simulink subsystem "original"  (R2025b)
settings: Solver=VariableStepAuto  StartTime=0.0  StopTime=10.0  RelTol=1e-3
settings Model: Creator=sanborkl  LastModifiedBy=sanborkl

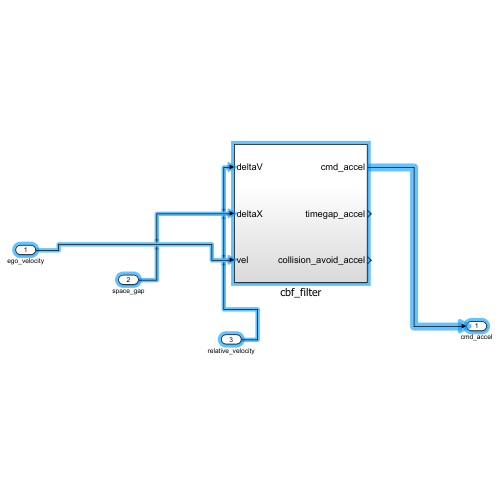
[thumbnail: Simulink's stored preview of the top-level diagram]
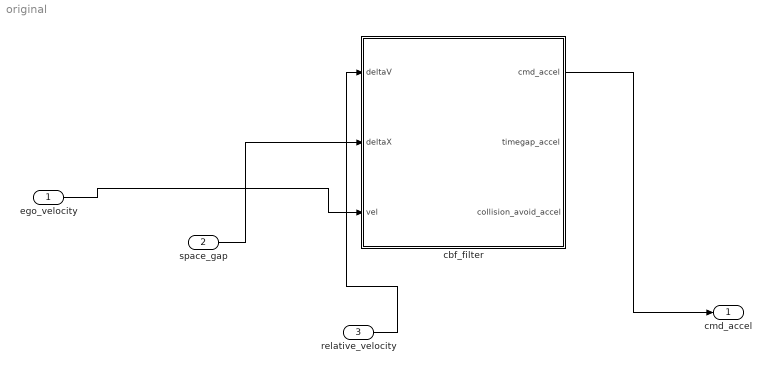
== system original ==
  ego_velocity : Inport
  space_gap : Inport  Port=2
  relative_velocity : Inport  Port=3
  cbf_filter : Subsystem
  cmd_accel : Outport
  wires:
  relative_velocity/1 -> cbf_filter/1(deltaV)
  ego_velocity/1 -> cbf_filter/3(vel)
  space_gap/1 -> cbf_filter/2(deltaX)
  cbf_filter/1(cmd_accel) -> cmd_accel/1

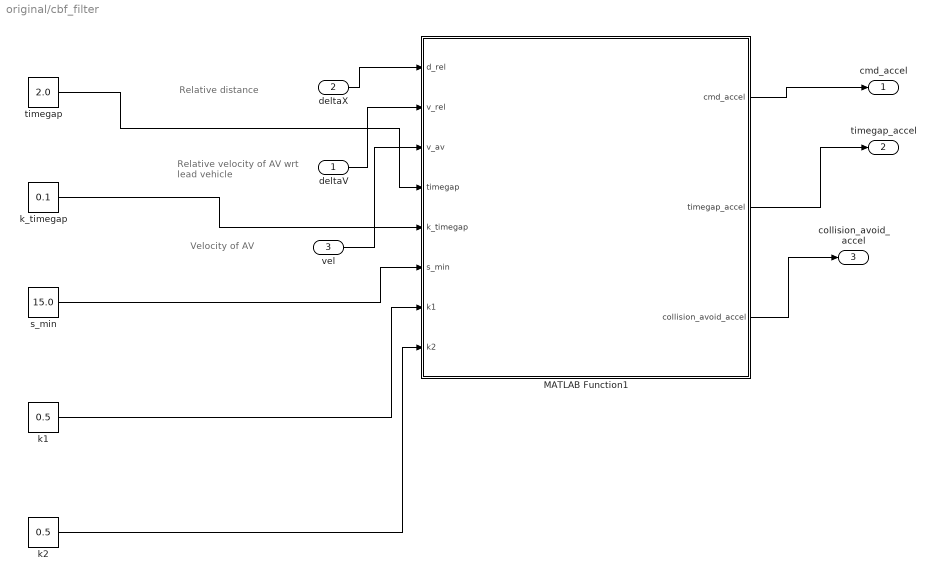
== system original/cbf_filter ==
  note: Velocity of AV
  note: Relative velocity of
      | AV wrt lead vehicle
  note: Relative distance
  deltaV : Inport
  deltaX : Inport  Port=2
  vel : Inport  Port=3
  MATLAB Function1 : MATLAB Function  TreatAsAtomicUnit=on
  k1 : Constant  Value=0.5
  k2 : Constant  Value=0.5
  k_timegap : Constant  Value=0.1
  s_min : Constant  Value=15.0
  timegap : Constant  Value=2.0
  cmd_accel : Outport
  timegap_accel : Outport  Port=2
  collision_avoid_accel : Outport  Port=3
  wires:
  k1/1 -> MATLAB Function1/7(k1)
  timegap/1 -> MATLAB Function1/4(timegap)
  k_timegap/1 -> MATLAB Function1/5(k_timegap)
  s_min/1 -> MATLAB Function1/6(s_min)
  MATLAB Function1/2(timegap_accel) -> timegap_accel/1
  MATLAB Function1/1(cmd_accel) -> cmd_accel/1
  vel/1 -> MATLAB Function1/3(v_av)
  deltaV/1 -> MATLAB Function1/2(v_rel)
  deltaX/1 -> MATLAB Function1/1(d_rel)
  k2/1 -> MATLAB Function1/8(k2)
  MATLAB Function1/3(collision_avoid_accel) -> collision_avoid_accel/1

== matlab function original/cbf_filter/MATLAB Function1 ==
  data: cmd_accel output; d_rel input; v_rel input; v_av input; timegap input; timegap_accel output; collision_avoid_accel output; k_timegap input; s_min input; k1 input; k2 input
function [cmd_accel, timegap_accel, collision_avoid_accel]= fcn(d_rel,v_rel,v_av, timegap,k_timegap,s_min,k1,k2)
%#codegen

% from the timegap filter function
% maybe make this gain a parameter later
% k = 0.1;
k = k_timegap;
%t_min = 2.0;
t_min = timegap;
timegap_accel = (1/t_min)*v_rel + (k/t_min)*(d_rel - t_min*v_av - s_min);

% from collision-avoid filter function
% a potential parameter - read into the fcn now
% s_min = 15.0;
% a potential parameter - read into the fcn now
% k1 = 0.5;
% a potential parameter - read into the fcn now
% k2 = 0.5;
%a_max = a_l + (k1+k2)*(delta_v) + (k1*k2)*(s-s_min);
% simplification TODO this is maybe dangerous so need to confirm
a_l = 0;
collision_avoid_accel = a_l + (k1+k2)*(v_rel) + (k1*k2)*(d_rel-s_min);

% now put these together
% 	 tg_accel = time_gap_filter(v,s,delta_v)
% 	 ca_accel = collision_avoid_filter(s,delta_v,a_l)
% 	 return min([tg_accel,ca_accel])
% TODO make max/min acceleration parameters.
% cmd_accel = min(1.5,max(-3.0,min(timegap_accel,collision_avoid_accel)));
cmd_accel = min(timegap_accel,collision_avoid_accel);
